simulink model "Fourvehiclecontinuous"  (R2022b)
settings: Solver=VariableStepAuto  StartTime=0.0  StopTime=10.0  RelTol=1e-3
values from neighbouring files (symbols this model uses):
  A = [0 1 0 0 0 0 0 0 ... (first row only)    [fourcarscontinuos.m]
  B = [0 0 0 0 ... (first row only)    [fourcarscontinuos.m]
  C = [1 -1 0 0 0 0 0 0 ... (first row only)    [fourcarscontinuos.m]
undefined symbols (not defined in the file or in its folder): L, U
libraries: simulink x2
settings Model: Creator=Hp Business  LastModifiedBy=Hp Business

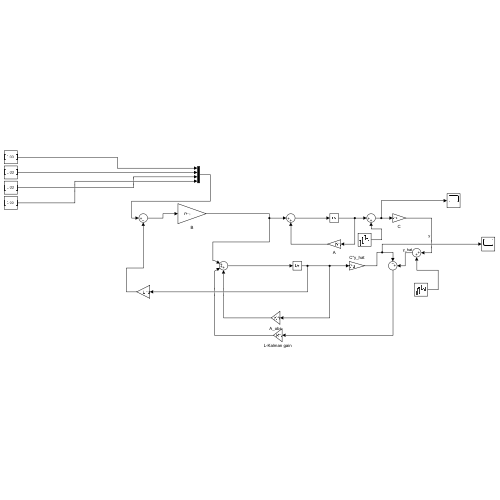
[thumbnail: Simulink's stored preview of the top-level diagram]
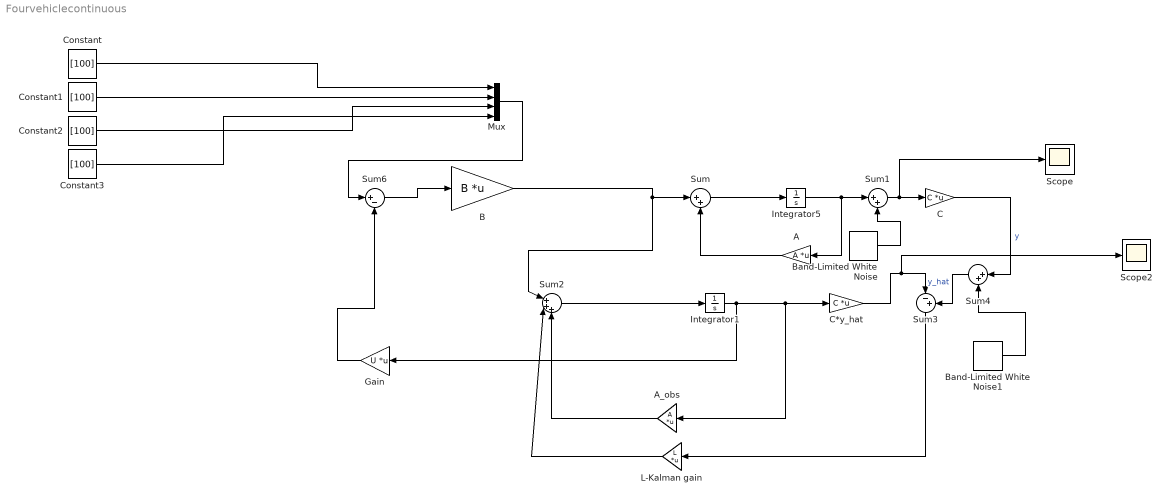
== system Fourvehiclecontinuous ==
  A : Gain  Gain=A  Multiplication=Matrix(K*u)
  A_obs : Gain  Gain=A  Multiplication=Matrix(K*u)
  B : Gain  Gain=B  Multiplication=Matrix(K*u)
  Band-Limited White Noise : simulink/Sources/Band-Limited White Noise  Cov=[1.1]  Ts=0.1  seed=[23341]
  Band-Limited White Noise1 : simulink/Sources/Band-Limited White Noise  Cov=[0.1]  Ts=0.1  seed=[23341]
  C : Gain  Gain=C  Multiplication=Matrix(K*u)
  C*y_hat : Gain  Gain=C  Multiplication=Matrix(K*u)
  Constant{,1..3} (4 alike) : Constant  Value=[100]
  Gain : Gain  Gain=U  Multiplication=Matrix(K*u)
  Integrator1 : Integrator
  Integrator5 : Integrator
  L-Kalman gain : Gain  Gain=L  Multiplication=Matrix(K*u)
  Mux : Mux
  Scope : Scope
  Scope2 : Scope
  Sum : Sum  Inputs=|++
  Sum1 : Sum  Inputs=|++
  Sum2 : Sum  Inputs=|+++
  Sum3 : Sum  Inputs=|-+
  Sum4 : Sum  Inputs=|++
  Sum6 : Sum  Inputs=|+-
  wires:
  Sum2/1 -> Integrator1/1
  B/1 -> Sum2/1, Sum/1
  Sum/1 -> Integrator5/1
  Integrator5/1 -> Sum1/1, A/1
  A/1 -> Sum/2
  C/1 -> Sum4/1  "y"
  Sum3/1 -> L-Kalman gain/1
  C*y_hat/1 -> Scope2/1, Sum3/1
  Integrator1/1 -> Gain/1, A_obs/1, C*y_hat/1
  A_obs/1 -> Sum2/3
  L-Kalman gain/1 -> Sum2/2
  Gain/1 -> Sum6/2
  Sum1/1 -> Scope/1, C/1
  Band-Limited White Noise/1 -> Sum1/2
  Band-Limited White Noise1/1 -> Sum4/2
  Sum4/1 -> Sum3/2  "y_hat"
  Mux/1 -> Sum6/1
  Sum6/1 -> B/1
  Constant2/1 -> Mux/3
  Constant1/1 -> Mux/2
  Constant/1 -> Mux/1
  Constant3/1 -> Mux/4
